simulink model "uklad1"  (R2021b)
settings: Solver=VariableStepAuto  StartTime=0.0  StopTime=10.0  RelTol=1e-3
settings Model: Creator=Student  LastModifiedBy=Student

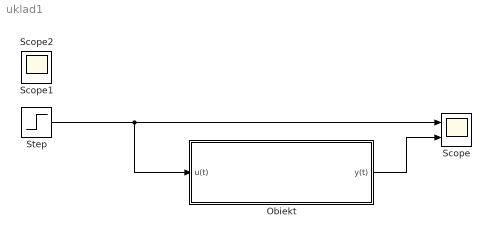
== system uklad1 ==
  Obiekt : Subsystem  mask{wn=1, zeta=0.5}
      mask prompts: wn "wn - częstotliwość drgań własnych"; zeta "zeta - współczynnik tłumienia"
  Scope : Scope  NumInputPorts=2
  Step : Step  Time=0  SampleTime=0
  Scope1 : Scope
  Scope2 : Scope
  wires:
  Step/1 -> Obiekt/1(u(t)), Scope/1
  Obiekt/1(y(t)) -> Scope/2

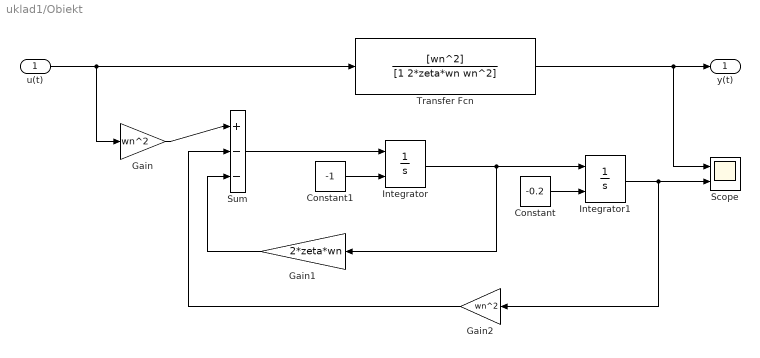
== system uklad1/Obiekt ==
  u(t) : Inport
  Constant : Constant  Value=-0.2
  Constant1 : Constant  Value=-1
  Gain : Gain  Gain=wn^2
  Gain1 : Gain  Gain=2*zeta*wn
  Gain2 : Gain  Gain=wn^2
  Integrator : Integrator  InitialConditionSource=external
  Integrator1 : Integrator  InitialConditionSource=external
  Scope : Scope  NumInputPorts=2
  Sum : Sum  Inputs=|+--
  Transfer Fcn : TransferFcn  Numerator=[wn^2]  Denominator=[1 2*zeta*wn wn^2]
  y(t) : Outport
  wires:
  Transfer Fcn/1 -> Scope/1, y(t)/1
  u(t)/1 -> Gain/1, Transfer Fcn/1
  Integrator1/1 -> Gain2/1, Scope/2
  Constant/1 -> Integrator1/2
  Integrator/1 -> Gain1/1, Integrator1/1
  Constant1/1 -> Integrator/2
  Sum/1 -> Integrator/1
  Gain/1 -> Sum/1
  Gain1/1 -> Sum/3
  Gain2/1 -> Sum/2
